simulink model "output_splitter"  (R2019a)
settings: Solver=VariableStepAuto  StartTime=0.0  StopTime=10000  FixedStep=1  RelTol=1e-3
InitFcn:
  | ini_cantonisim_distributed
undefined symbols (not defined in the file or in its folder): C1, C2
settings Model: Creator=Jacob  LastModifiedBy=Jacob
settings SolverCC: AlgebraicLoopSolver=LineSearch
settings DataIOCC: SaveOutput=off  SaveTime=off

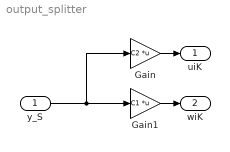
== system output_splitter ==
  y_S : Inport  OutDataTypeStr=double  PortDimensions=2  SampleTime=0
  Gain : Gain  Gain=C2  Multiplication=Matrix(K*u)
  Gain1 : Gain  Gain=C1  Multiplication=Matrix(K*u)
  uiK : Outport  OutDataTypeStr=double  PortDimensions=1  SampleTime=0
  wiK : Outport  Port=2  OutDataTypeStr=double  PortDimensions=1  SampleTime=0
  wires:
  y_S/1 -> Gain1/1, Gain/1
  Gain1/1 -> wiK/1
  Gain/1 -> uiK/1
